simulink model "WIP_mb_model"  (R2025b)
settings: Solver=ode23t  StartTime=0.0  StopTime=10.0  MaxStep=1e-3  RelTol=1e-3  AbsTol=1e-3
settings Model: Creator=upattacini  LastModifiedBy=upattacini
settings DataIOCC: SaveOutput=off  DSMLogging=off  SaveTime=off
settings ModelReferenceCC: UpdateModelReferenceTargets=Force

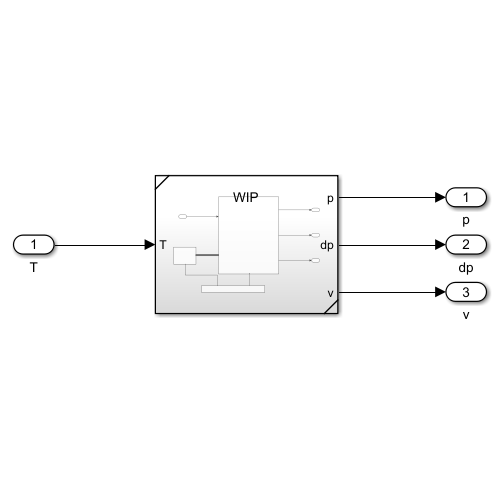
[thumbnail: Simulink's stored preview of the top-level diagram]
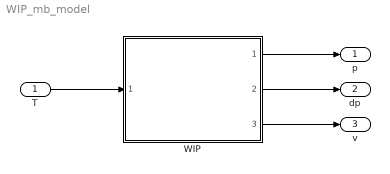
== system WIP_mb_model ==
  T : Inport
  WIP : Subsystem  ReferencedSubsystem=WIP
  p : Outport
  dp : Outport  Port=2
  v : Outport  Port=3
  wires:
  WIP/2 -> dp/1
  T/1 -> WIP/1
  WIP/3 -> v/1
  WIP/1 -> p/1
